simulink model "Taller"  (R2024a)
settings: Solver=VariableStepAuto  StartTime=0.0  StopTime=50  RelTol=1e-3
settings Model: Creator=EVJA_3  LastModifiedBy=camil
settings SolverCC: AlgebraicLoopSolver=TrustRegion
settings DataIOCC: ReturnWorkspaceOutputs=off
settings DebuggingCC: UnconnectedInputMsg=warning  UnconnectedOutputMsg=warning  UnconnectedLineMsg=warning  ArithmeticOperatorsInVariantConditions=warning
settings ModelReferenceCC: EnableRefExpFcnMdlSchedulingChecks=on
settings SFSimCC: SimUseLocalCustomCode=off  CustomCodeUndefinedFunction=UseInterfaceOnly
settings RTWCC: RTWUseLocalCustomCode=off  GPUComputeCapability=3.5

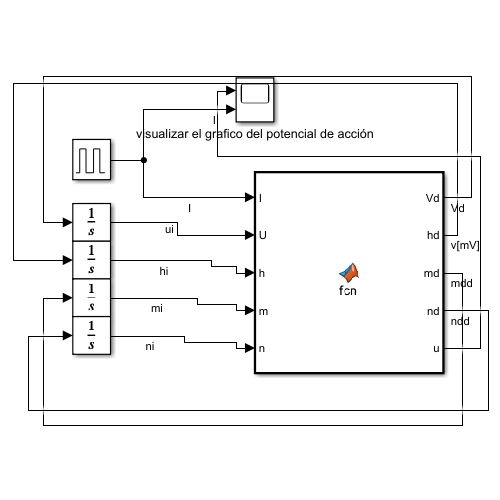
[thumbnail: Simulink's stored preview of the top-level diagram]
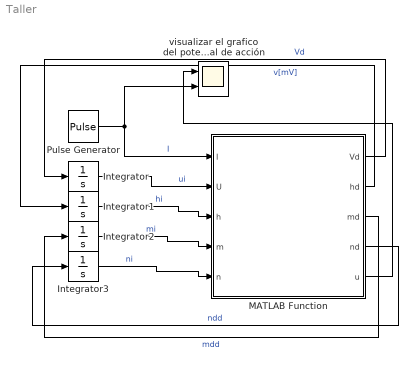
== system Taller ==
  Integrator : Integrator  InitialCondition=65
  Integrator1 : Integrator  InitialCondition=0.5
  Integrator2 : Integrator  InitialCondition=0.06
  Integrator3 : Integrator  InitialCondition=0.5
  MATLAB Function : MATLAB Function  TreatAsAtomicUnit=on
  Pulse Generator : DiscretePulseGenerator  PulseType=Time based  Amplitude=50  Period=20  PulseWidth=25  PhaseDelay=5
  visualizar el grafico del potencial de acción : Scope  NumInputPorts=2
  wires:
  Integrator/1 -> MATLAB Function/2(U)  "ui"
  Integrator1/1 -> MATLAB Function/3(h)  "hi"
  Integrator2/1 -> MATLAB Function/4(m)  "mi"
  Integrator3/1 -> MATLAB Function/5(n)  "ni"
  Pulse Generator/1 -> MATLAB Function/1(I), visualizar el grafico del potencial de acción/2  "I"
  MATLAB Function/3(md) -> Integrator2/1  "mdd"
  MATLAB Function/4(nd) -> Integrator3/1  "ndd"
  MATLAB Function/1(Vd) -> Integrator/1  "Vd"
  MATLAB Function/2(hd) -> Integrator1/1  "v[mV]"
  MATLAB Function/5(u) -> visualizar el grafico del potencial de acción/1

== matlab function Taller/MATLAB Function ==
  data: I input; U input; Vd output; h input; m input; n input; hd output; md output; nd output; u output
function [Vd,hd,md,nd,u] = fcn(I,U,h,m,n)
% constantes

C=1;%unidades de medida micros, capacitancia de la membrana 
gLn=0.3;%milisvalores de conductancia normales para otros 

VL=-55;%milis,potencial de accion de otros iones 
VK=-70;%milis, potencial de accion del potasio intra celular 
VNa=40;%milis, potencial de accion del sodio  extra celular  

gKn=36;%milis, valores de de conductacia normal del potasio 
gNan=120;%milis,valores de de conductacia normal del sodio

Ueq=-65;%milis, potencial de equilibrio de la membrana 
u=U-Ueq;%milis, potencial de la membrana en cualquier momento menos potencial de equilibrio de la membrana

% h , m, n
ah=0.07*exp(u/-20);%alpha de h 
bh=1/(exp(3-0.1*(u))+1);%beta de h


am=(2.5-0.1*(u))/(exp(2.5-0.1*(u))-1);%alpha de m
bm=4*exp(u/-18);%beta de m


an=(0.1-0.01*(u))/(exp(1-0.1*(u))-1);%alpha de n
bn=0.125*exp(u/-80);%beta de n

% Integrales  

gNa=gNan*h*m^3;
gK=gKn*n^4;

%Calculando las corrientes
INa=gNa*(u-VNa);
IK=gK*(u-VK);
IL=gLn*(u-VL);
%Corriente total de los inoes 
F=INa+IK+IL;

%funciones de salida
Vd = (-F+I)/C;
hd = ah*(1-h)-bh*h;
md = am*(1-m)-bm*m;
nd = an*(1-n)-bn*n;
